simulink model "polyinterp_2_"  (Simulink 7.8)
settings: Solver=ode45  StartTime=0.0  StopTime=2.0  RelTol=1e-3
values from neighbouring files (symbols this model uses):
  h = firpm(64,f,m)    [CFIR_1.m]    (also in adapt_filter1.m = adaptfilt.lms(ni,mu); adapt_filter2.m = adaptfilt.blms(ni,mu,1,36); adaptiv_2.m = [1 2 3 4 5 6 7 8 9 10]; adaptiv_3.m = [1 2 3 4 5 6 7 8 9 10])
  Ts = 1/fs    (= 6.25e-05)    [G722_1.m]    (also in adaptiv_2.m = 0.001; adaptiv_3.m = 0.001; adaptiv_4.m = 0.001; adaptiv_5.m = 0.001)
undefined symbols (not defined in the file or in its folder): g
libraries: dspsigops x2, dspobslib x1
settings Model: Creator=svenhoffmann  LastModifiedBy=josef  ExtModeAutoUpdateStatusClock=off
settings DataIOCC: SignalLoggingName=sigsOut
settings OptimizationCC: InitFltsAndDblsToZero=on
settings DebuggingCC: SaveWithParameterizedLinksMsg=none  SignalResolutionControl=TryResolveAllWithWarning  SolverPrmCheckMsg=none  MultiTaskDSMMsg=warning  MultiTaskCondExecSysMsg=none  FcnCallInpInsideContextMsg=Use local settings  StrictBusMsg=None
settings HardwareCC: TargetUnknown=on
settings RTWCC: IncludeERTFirstTime=on
settings GRTTargetCC: TargetFcnLib=ansi_tfl_tmw.mat

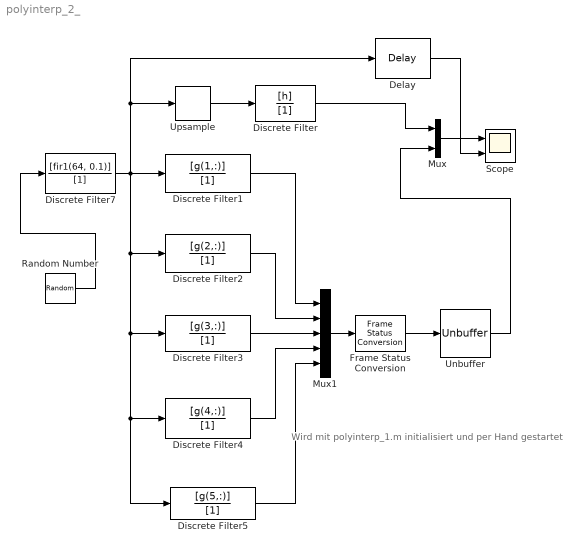
== system polyinterp_2_ ==
  note: Wird mit polyinterp_1.m
      | initialisiert und per Hand
      | gestartet
  Delay : dspsigops/Delay  InputProcessing=Inherited (this choice will be removed - see release notes)  dly_unit=Samples  delay=13  ic_detail=off  dif_ic_for_ch=off  dif_ic_for_dly=off  ic=0  reset_popup=None
  Discrete Filter : DiscreteFilter  Numerator=[h]  Denominator=[1]  SampleTime=Ts/5
  Discrete Filter1 : DiscreteFilter  Numerator=[g(1,:)]  Denominator=[1]  SampleTime=Ts
  Discrete Filter2 : DiscreteFilter  Numerator=[g(2,:)]  Denominator=[1]  SampleTime=Ts
  Discrete Filter3 : DiscreteFilter  Numerator=[g(3,:)]  Denominator=[1]  SampleTime=Ts
  Discrete Filter4 : DiscreteFilter  Numerator=[g(4,:)]  Denominator=[1]  SampleTime=Ts
  Discrete Filter5 : DiscreteFilter  Numerator=[g(5,:)]  Denominator=[1]  SampleTime=Ts
  Discrete Filter7 : DiscreteFilter  Numerator=[fir1(64, 0.1)]  Denominator=[1]  SampleTime=Ts
  Frame Status Conversion : dspobslib/Frame Status Conversion  growRefPort=off  outframe=Frame-based
  Mux : Mux  Inputs=2
  Mux1 : Mux  Inputs=5
  Random Number : RandomNumber  SampleTime=Ts
  Scope : Scope  NumInputPorts=2
      settings: YMin=-0.3~-15  YMax=0.35~12.5
  Unbuffer : Unbuffer
  Upsample : dspsigops/Upsample  N=5  phase=0  InputProcessing=Inherited (this choice will be removed - see release notes)  RateOptions=Allow multirate processing  ic=0  mode=Unused parameter value
  wires:
  Random Number/1 -> Discrete Filter7/1
  Discrete Filter/1 -> Mux/1
  Discrete Filter1/1 -> Mux1/1
  Discrete Filter3/1 -> Mux1/3
  Mux/1 -> Scope/1
  Upsample/1 -> Discrete Filter/1
  Discrete Filter7/1 -> Discrete Filter1/1, Upsample/1, Delay/1, Discrete Filter2/1, Discrete Filter3/1, Discrete Filter4/1, Discrete Filter5/1
  Discrete Filter2/1 -> Mux1/2
  Discrete Filter4/1 -> Mux1/4
  Discrete Filter5/1 -> Mux1/5
  Mux1/1 -> Frame Status Conversion/1
  Unbuffer/1 -> Mux/2
  Frame Status Conversion/1 -> Unbuffer/1
  Delay/1 -> Scope/2
